simulink model "ultimointento2"  (Simulink 7.9)
settings: Solver=ode45  StartTime=0.0  StopTime=150  RelTol=1e-3
settings Model: Creator=Miguel Faggioni  LastModifiedBy=Miguel Faggioni
settings DataIOCC: TimeSaveName=t  OutputSaveName=sal

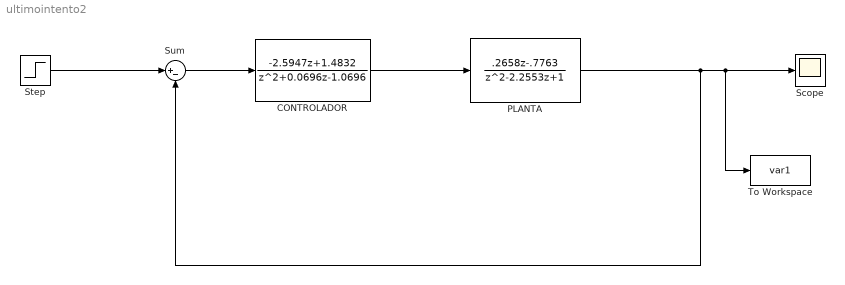
== system ultimointento2 ==
  CONTROLADOR : DiscreteTransferFcn  Numerator=[-2.5947 1.4832]  Denominator=[1 0.0696 -1.0696]
  PLANTA : DiscreteTransferFcn  Numerator=[.2658 -.7763]  Denominator=[1 -2.2553 1]
  Scope : Scope
      settings: TimeRange=150  YMin=-2e+307  YMax=5.000000000000001e+306
  Step : Step  Time=0  SampleTime=.25
  Sum : Sum  Inputs=|+-
  To Workspace : ToWorkspace  VariableName=var1  SampleTime=-1  SaveFormat=Timeseries
  wires:
  Sum/1 -> CONTROLADOR/1
  CONTROLADOR/1 -> PLANTA/1
  PLANTA/1 -> Sum/2, Scope/1, To Workspace/1
  Step/1 -> Sum/1
